simulink model "transformation_between_coordinate_frames"  (R2022a)
settings: Solver=VariableStepAuto  StartTime=0.0  StopTime=0.5  RelTol=1e-3
model workspace: external: MATLAB File D:\Simulink\Study\transformation_between_coordinate_frames_Parameters.m (data not in the file)
values from neighbouring files (symbols this model uses):
  B = 0.008    [transformation_between_coordinate_frames_Parameters.m]
  J = 0.001    [transformation_between_coordinate_frames_Parameters.m]
  Pn = 4    [transformation_between_coordinate_frames_Parameters.m]
  R = 2.875    [transformation_between_coordinate_frames_Parameters.m]
  V = 100    [transformation_between_coordinate_frames_Parameters.m]
undefined symbols (not defined in the file or in its folder): DiscIntNeverNeededParam
libraries: spsControlledVoltageSourceLib x3, spsGroundLib x1, spsPermanentMagnetSynchronousMachineLib x1, spspowerguiLib x1
settings Model: Creator=123  LastModifiedBy=123

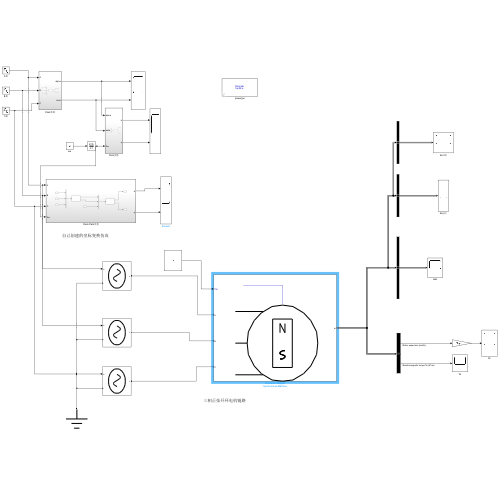
[thumbnail: Simulink's stored preview of the top-level diagram]
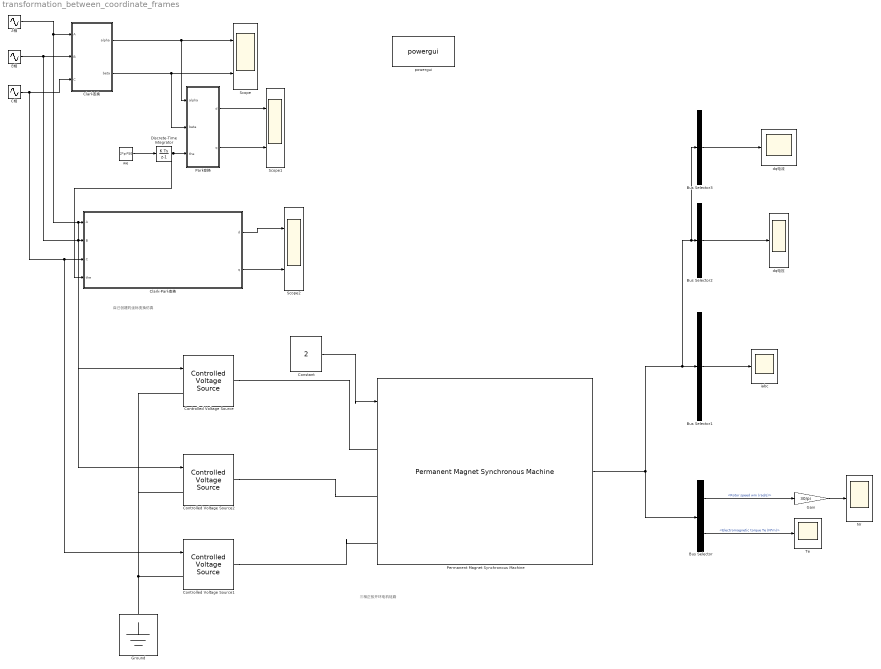
== system transformation_between_coordinate_frames ==
  note: 三相正弦开环电机链路
  note: 自己创建的坐标变换仿真
  A相 : Sin  Amplitude=100  Frequency=2*pi*50  SampleTime=2e-5
  Bus Selector : BusSelector  OutputSignals=Rotor speed wm (rad/s),Electromagnetic torque Te (N*m)
  Bus Selector1 : BusSelector  OutputSignals=Stator current is_a (A),Stator current is_b (A),Stator current is_c (A)  OutputAsBus=on
  Bus Selector2 : BusSelector  OutputSignals=Stator voltage Vs_d (V),Stator voltage Vs_q (V)  OutputAsBus=on
  Bus Selector3 : BusSelector  OutputSignals=Stator current is_q (A),Stator current is_d (A)  OutputAsBus=on
  B相 : Sin  Amplitude=100  Frequency=2*pi*50  Phase=-pi*2/3  SampleTime=2e-5
  Clark-Park变换 : Subsystem
  Clark变换 : Subsystem
  Constant : Constant  Value=2
  Controlled Voltage Source : spsControlledVoltageSourceLib/Controlled Voltage Source  Initialize=on  Source_Type=AC  Amplitude=0  Phase=0  Frequency=0  Measurements=None
  Controlled Voltage Source1 : spsControlledVoltageSourceLib/Controlled Voltage Source  Initialize=on  Source_Type=AC  Amplitude=0  Phase=0  Frequency=0  Measurements=None
  Controlled Voltage Source2 : spsControlledVoltageSourceLib/Controlled Voltage Source  Initialize=on  Source_Type=AC  Amplitude=0  Phase=0  Frequency=0  Measurements=None
  C相 : Sin  Amplitude=100  Frequency=2*pi*50  Phase=pi*2/3  SampleTime=2e-5
  Discrete-Time Integrator : DiscreteIntegrator  SampleTime=-1  ICPrevOutput=DiscIntNeverNeededParam  ICPrevScaledInput=DiscIntNeverNeededParam
  Gain : Gain  Gain=30/pi
  Ground : spsGroundLib/Ground  LConnTagsString=a
  Nr : Scope
  Park变换 : Subsystem
  Permanent Magnet Synchronous Machine : spsPermanentMagnetSynchronousMachineLib/Permanent Magnet Synchronous Machine  NbPhases=3  FluxDistribution=Sinusoidal  RotorType=Round  MechanicalLoad=Torque Tm  PresetModel=No  ShowDetailedParameters=on  MeasurementBus=off  Resistance=R  Inductance=8.5e-3  dqInductances=[8.5e-3,8.5e-3]  La=Ld  MachineConstant=Flux linkage established by magnets (V.s)  Flux=flux  VoltageCst=126.966  TorqueCst=1.05  Flat=120  Mechanical=[J B Pn 0]  PolePairs=4  InitialConditions=[0,0, 0,0]  InitialConditions5ph=[0 0 0 0 0 0]  RefAngle=Aligned with phase A axis (original Park)  IterativeDiscreteModel=Trapezoidal non iterative  TsBlock=-1  TsPowergui=0
  Scope : Scope  NumInputPorts=2
  Scope1 : Scope  NumInputPorts=2
  Scope2 : Scope  NumInputPorts=2
  Te : Scope
  dq电压 : Scope
  dq电流 : Scope
  iabc : Scope
  powergui : spspowerguiLib/powergui  Priority=1  SimulationMode=Discrete  SampleTime=5e-6  frequency=60  Iterations=50  frequencyindice=0  Pbase=100e6  ErrMax=1e-4  UnitsV=kV  UnitsW=MW  buscounter=0  FunctionMessages=off  echomessages=off  EnableUseOfTLC=off  CurrentSourceSwitches=off  DisableSnubberDevices=off  DisableRonSwitches=off  DisableVfSwitches=off  DisplayEquations=off  AutomaticDiscreteSolvers=off  SolverType=Tustin/Backward Euler (TBE)  Interpol=off  ExternalGateDelay=off  methode=off  Ts=100  x0status=blocks  SPID=on  SwTol=0  HookPort=off  NonlinearTolerance=1e-4  nMaxIteration=100  ContinueOnMaxIteration=off  RestoreLinks=warning  ResistiveCurrentMeasurement=off  Frange=[0:2:500]  Ylog=off  Xlog=on  ShowGrid=off  save=off  variable=ZData  structure=0  ZoomFFT=off  StartTime=0.0  cycles=1  DisplayStyle=1  fundamental=60  FreqAxis=off  MaxFrequency=1000  frequencyindicesteady=1  RmsSteady=1  display=off
  we : Constant  Value=2*pi*50  SampleTime=2e-5
  wires:
  A相/1 -> Clark变换/1(A), Controlled Voltage Source/1, Clark-Park变换/1(A)
  B相/1 -> Clark变换/2(B), Controlled Voltage Source2/1, Clark-Park变换/2(B)
  C相/1 -> Clark变换/3(C), Clark-Park变换/3(C), Controlled Voltage Source1/1
  Clark变换/1(alpha) -> Park变换/1(alpha), Scope/1
  Clark变换/2(beta) -> Scope/2, Park变换/2(beta)
  we/1 -> Discrete-Time Integrator/1
  Discrete-Time Integrator/1 -> Clark-Park变换/4(the), Park变换/3(the)
  Park变换/1(d) -> Scope1/1
  Park变换/2(q) -> Scope1/2
  Clark-Park变换/1(d) -> Scope2/1
  Clark-Park变换/2(q) -> Scope2/2
  Constant/1 -> Permanent Magnet Synchronous Machine/1
  Permanent Magnet Synchronous Machine/1 -> Bus Selector1/1, Bus Selector3/1, Bus Selector2/1, Bus Selector/1
  Bus Selector1/1 -> iabc/1
  Gain/1 -> Nr/1
  Bus Selector/1 -> Gain/1  "<Rotor speed wm (rad/s)>"
  Bus Selector/2 -> Te/1  "<Electromagnetic torque Te (N*m)>"
  Bus Selector2/1 -> dq电压/1
  Bus Selector3/1 -> dq电流/1
  connections:
  Controlled Voltage Source/RConn1 -- Permanent Magnet Synchronous Machine/LConn1
  Controlled Voltage Source2/RConn1 -- Permanent Magnet Synchronous Machine/LConn2
  Controlled Voltage Source1/RConn1 -- Permanent Magnet Synchronous Machine/LConn3
  Controlled Voltage Source1/LConn1 -- Controlled Voltage Source/LConn1 -- Controlled Voltage Source2/LConn1 -- Ground/LConn1

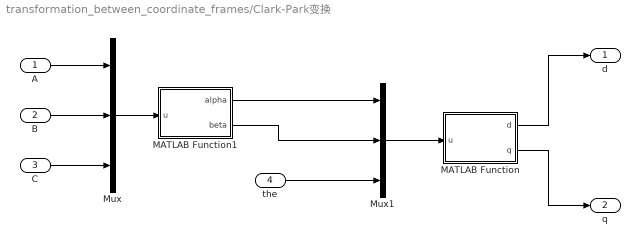
== system transformation_between_coordinate_frames/Clark-Park变换 ==
  A : Inport
  B : Inport  Port=2
  C : Inport  Port=3
  the : Inport  Port=4
  MATLAB Function : MATLAB Function  TreatAsAtomicUnit=on
  MATLAB Function1 : MATLAB Function  TreatAsAtomicUnit=on
  Mux : Mux  Inputs=3
  Mux1 : Mux  Inputs=3
  d : Outport
  q : Outport  Port=2
  wires:
  A/1 -> Mux/1
  B/1 -> Mux/2
  Mux/1 -> MATLAB Function1/1(u)
  C/1 -> Mux/3
  MATLAB Function/2(q) -> q/1
  MATLAB Function/1(d) -> d/1
  Mux1/1 -> MATLAB Function/1(u)
  MATLAB Function1/1(alpha) -> Mux1/1
  MATLAB Function1/2(beta) -> Mux1/2
  the/1 -> Mux1/3

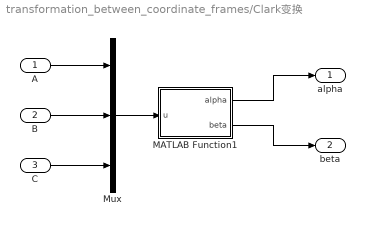
== system transformation_between_coordinate_frames/Clark变换 ==
  A : Inport
  B : Inport  Port=2
  C : Inport  Port=3
  MATLAB Function1 : MATLAB Function  TreatAsAtomicUnit=on
  Mux : Mux  Inputs=3
  alpha : Outport
  beta : Outport  Port=2
  wires:
  A/1 -> Mux/1
  B/1 -> Mux/2
  C/1 -> Mux/3
  Mux/1 -> MATLAB Function1/1(u)
  MATLAB Function1/1(alpha) -> alpha/1
  MATLAB Function1/2(beta) -> beta/1

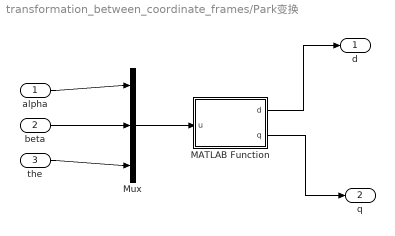
== system transformation_between_coordinate_frames/Park变换 ==
  alpha : Inport
  beta : Inport  Port=2
  the : Inport  Port=3
  MATLAB Function : MATLAB Function  TreatAsAtomicUnit=on
  Mux : Mux  Inputs=3
  d : Outport
  q : Outport  Port=2
  wires:
  alpha/1 -> Mux/1
  beta/1 -> Mux/2
  the/1 -> Mux/3
  Mux/1 -> MATLAB Function/1(u)
  MATLAB Function/1(d) -> d/1
  MATLAB Function/2(q) -> q/1

== matlab function transformation_between_coordinate_frames/Park变换/MATLAB Function ==
  data: u input; d output; q output
function [d,q]  = fcn(u)

d = u(1)*cos(u(3))+u(2)*sin(u(3));
q = -u(1)*sin(u(3))+u(2)*cos(u(3));

end

== matlab function transformation_between_coordinate_frames/Clark-Park变换/MATLAB Function1 ==
  data: u input; alpha output; beta output
function [alpha, beta] = fcn(u)

alpha = (u(1)-0.5*(u(2)+u(3)))*2/3;
beta  = sqrt(3)/2*(u(2)-u(3))*2/3;

end

== matlab function transformation_between_coordinate_frames/Clark-Park变换/MATLAB Function ==
  data: u input; d output; q output
function [d,q]  = fcn(u)

d = u(1)*cos(u(3))+u(2)*sin(u(3));
q = -u(1)*sin(u(3))+u(2)*cos(u(3));

end

== matlab function transformation_between_coordinate_frames/Clark变换/MATLAB Function1 ==
  data: u input; alpha output; beta output
function [alpha, beta] = fcn(u)

alpha = (u(1)-0.5*(u(2)+u(3)))*2/3;
beta  = sqrt(3)/2*(u(2)-u(3))*2/3;

end
